simulink model "reactor_feedback_full_state"  (Simulink 10.2)
settings: Solver=ode15s  StartTime=0.0  StopTime=100  RelTol=1e-6  EnableMultiTasking=on
values from neighbouring files (symbols this model uses):
  C_A_steady = x_ss(1)    [assignment_q2.m]
  C_B_steady = x_ss(2)    [assignment_q2.m]
  K = place(A_linearized, B_linearized, new_eig_values_K)    [assignment_q2.m]
  T_J_steady = x_ss(4)    [assignment_q2.m]
  T_R_steady = x_ss(3)    [assignment_q2.m]
  u_s = [Fr_ss Qj_ss]    [assignment_q2.m]
settings Model: Creator=LemoineR  LastModifiedBy=mbatu
settings DataIOCC: LimitDataPoints=on
settings OptimizationCC: ExpressionDepthLimit=2147483647
settings DebuggingCC: SolverPrmCheckMsg=warning  StateNameClashWarn=warning

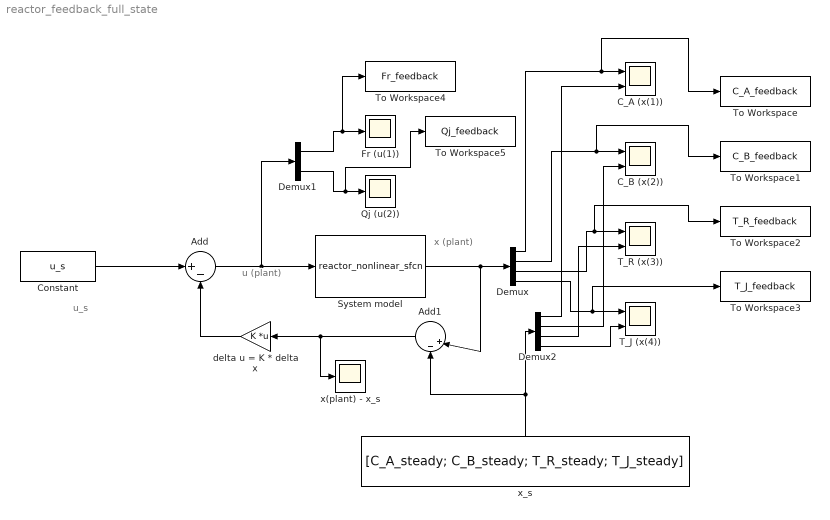
== system reactor_feedback_full_state ==
  note: u_s
  note: u (plant)
  note: x (plant)
  Add : Sum  Inputs=|+-
  Add1 : Sum  Inputs=||+-
  C_A (x(1)) : Scope  NumInputPorts=2
  C_B (x(2)) : Scope  NumInputPorts=2
  Constant : Constant  Value=u_s
  Demux : Demux
  Demux1 : Demux  Outputs=2
  Demux2 : Demux
  Fr (u(1)) : Scope
  Qj (u(2)) : Scope
  System model : S-Function  FunctionName=reactor_nonlinear_sfcn  SFunctionDeploymentMode=off  EnableBusSupport=off
  T_J (x(4)) : Scope  NumInputPorts=2
  T_R (x(3)) : Scope  NumInputPorts=2
  To Workspace : ToWorkspace  VariableName=C_A_feedback  SampleTime=-1
  To Workspace1 : ToWorkspace  VariableName=C_B_feedback  SampleTime=-1
  To Workspace2 : ToWorkspace  VariableName=T_R_feedback  SampleTime=-1
  To Workspace3 : ToWorkspace  VariableName=T_J_feedback  SampleTime=-1
  To Workspace4 : ToWorkspace  VariableName=Fr_feedback  SampleTime=-1
  To Workspace5 : ToWorkspace  VariableName=Qj_feedback  SampleTime=-1
  delta u = K * delta x : Gain  Gain=K  Multiplication=Matrix(K*u)
  x(plant) - x_s : Scope
  x_s : Constant  Value=[C_A_steady; C_B_steady; T_R_steady; T_J_steady]
  wires:
  System model/1 -> Add1/1, Demux/1
  Constant/1 -> Add/1
  delta u = K * delta x/1 -> Add/2
  x_s/1 -> Demux2/1, Add1/2
  Add1/1 -> x(plant) - x_s/1, delta u = K * delta x/1
  Demux1/1 -> To Workspace4/1, Fr (u(1))/1
  Demux1/2 -> To Workspace5/1, Qj (u(2))/1
  Add/1 -> Demux1/1, System model/1
  Demux/1 -> To Workspace/1, C_A (x(1))/1
  Demux/2 -> To Workspace1/1, C_B (x(2))/1
  Demux/3 -> To Workspace2/1, T_R (x(3))/1
  Demux/4 -> To Workspace3/1, T_J (x(4))/1
  Demux2/1 -> C_A (x(1))/2
  Demux2/2 -> C_B (x(2))/2
  Demux2/3 -> T_R (x(3))/2
  Demux2/4 -> T_J (x(4))/2
